simulink model "Project (2)"  (R2025b)
settings: Solver=VariableStepAuto  StartTime=0.0  StopTime=10.0  RelTol=1e-3

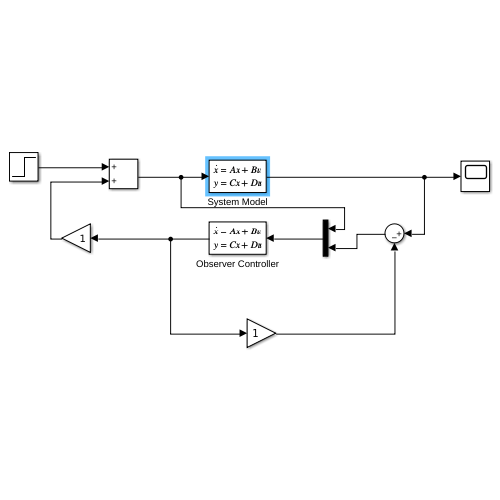
[thumbnail: Simulink's stored preview of the top-level diagram]
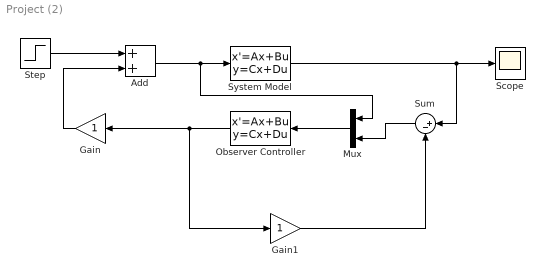
== system Project (2) ==
  Add : Sum
  Gain : Gain
  Gain1 : Gain
  Mux : Mux  Inputs=2
  Observer Controller : StateSpace  InitialCondition=0
  Scope : Scope
  Step : Step  SampleTime=0
  Sum : Sum  Inputs=|+-
  System Model : StateSpace  A=|  B=|  C=[1 0 1]  D=0  InitialCondition=0
      A=|
      | [-0.313  56.7   0
      | ; -0.0139  -0.426 0
      |  ; 0  56.7   0]
      B=|
      | [0.232;
      |  0.0203;
      |  0]
  wires:
  Step/1 -> Add/1
  Gain/1 -> Add/2
  Add/1 -> Mux/1, System Model/1
  Sum/1 -> Mux/2
  System Model/1 -> Sum/1, Scope/1
  Mux/1 -> Observer Controller/1
  Observer Controller/1 -> Gain1/1, Gain/1
  Gain1/1 -> Sum/2
